simulink model "ese1_massa"  (Simulink 7.5)
settings: Solver=ode45  StartTime=0.0  StopTime=20  RelTol=1e-3
values from neighbouring files (symbols this model uses):
  A = [0 1;-k/m -b/m]    [EsercizioMassaMollaSmorzatore.m]    (also in guida_comandi.m = 2; serb_continuo.m = [-k1 0; k1 -k2]; serbatoi.m = [-k1/s1 0;k1/s2 -k2/s2])
  B = [0;1/m]    [EsercizioMassaMollaSmorzatore.m]    (also in guida_comandi.m = [1 2 3;4 10 6]; serb_continuo.m = [1; 0]; serbatoi.m = [1/s1;0])
  C = [1 0]    [EsercizioMassaMollaSmorzatore.m]    (also in guida_comandi.m = [6 8 10;4 5 1]; serb_continuo.m = [0 k2]; serbatoi.m = [0 k2])
  D = 0    [EsercizioMassaMollaSmorzatore.m]    (also in serb_continuo.m; serbatoi.m)
  ueq = 2    [EsercizioMassaMollaSmorzatore.m]    (also in serb_continuo.m = 1; serbatoi.m = 1)
  x0 = [0 0]'    [EsercizioMassaMollaSmorzatore.m]    (also in serb_continuo.m = [1;1]; serbatoi.m = [1 1]')
libraries: simulink x1
settings Model: Creator=professore  LastModifiedBy=professore

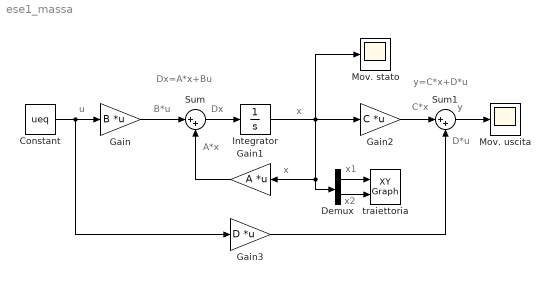
== system ese1_massa ==
  note: Dx=A*x+Bu
  note: y=C*x+D*u
  note: A*x
  note: B*u
  note: u
  note: x
  note: Dx
  note: x
  note: C*x
  note: D*u
  note: y
  note: x1
  note: x2
  Constant : Constant  Value=ueq  OutDataType=fixdt(1, 16)  OutScaling=2^0
  Demux : Demux  Outputs=2
  Gain : Gain  Gain=B  Multiplication=Matrix(K*u)  ParameterDataType=fixdt(1, 16)  ParameterScaling=2^0  OutDataType=fixdt(1, 16)  OutScaling=2^0
  Gain1 : Gain  Gain=A  Multiplication=Matrix(K*u)  ParameterDataType=fixdt(1, 16)  ParameterScaling=2^0  OutDataType=fixdt(1, 16)  OutScaling=2^0
  Gain2 : Gain  Gain=C  Multiplication=Matrix(K*u)  ParameterDataType=fixdt(1, 16)  ParameterScaling=2^0  OutDataType=fixdt(1, 16)  OutScaling=2^0
  Gain3 : Gain  Gain=D  Multiplication=Matrix(K*u)  ParameterDataType=fixdt(1, 16)  ParameterScaling=2^0  OutDataType=fixdt(1, 16)  OutScaling=2^0
  Integrator : Integrator  InitialCondition=x0
  Mov. stato : Scope
  Mov. uscita : Scope
  Sum : Sum  Inputs=|++  OutDataType=fixdt(1, 16)  OutScaling=2^0
  Sum1 : Sum  Inputs=|++  OutDataType=fixdt(1, 16)  OutScaling=2^0
  traiettoria : simulink/Sinks/XY Graph  SystemSampleTime=-1  xmin=0  xmax=8  ymin=0  ymax=2  st=-1
  wires:
  Gain/1 -> Sum/1
  Gain1/1 -> Sum/2
  Constant/1 -> Gain/1, Gain3/1
  Integrator/1 -> Gain2/1, Mov. stato/1, Gain1/1, Demux/1
  Sum/1 -> Integrator/1
  Gain2/1 -> Sum1/1
  Gain3/1 -> Sum1/2
  Sum1/1 -> Mov. uscita/1
  Demux/1 -> traiettoria/1
  Demux/2 -> traiettoria/2
